simulink model "Sim_Knickarmroboter_AndreasPaul"  (R2024a)
settings: Solver=VariableStepAuto  StartTime=0.0  StopTime=10.0  RelTol=1e-3
values from neighbouring files (symbols this model uses):
  F_s1 = 8.5e-4    (= 0.00085)    [Initialisierung_Kickarmroboter.m]
  F_s2 = 3.2e-4    (= 0.00032)    [Initialisierung_Kickarmroboter.m]
  g = 9.81    [Initialisierung_Kickarmroboter.m]
  I1 = 0.0309    [Initialisierung_Kickarmroboter.m]
  I2 = 0.0045    [Initialisierung_Kickarmroboter.m]
  l1 = 0.16    [Initialisierung_Kickarmroboter.m]
  l2 = 0.128    [Initialisierung_Kickarmroboter.m]
  m1 = 0.1817    [Initialisierung_Kickarmroboter.m]
  m2 = 0.0944    [Initialisierung_Kickarmroboter.m]
  mu_v1 = 3.843e-6    (= 3.843e-06)    [Initialisierung_Kickarmroboter.m]
  mu_v2 = 3.887e-6    (= 3.887e-06)    [Initialisierung_Kickarmroboter.m]
libraries: slpidlib x1
settings Model: Creator=apaul  LastModifiedBy=apaul

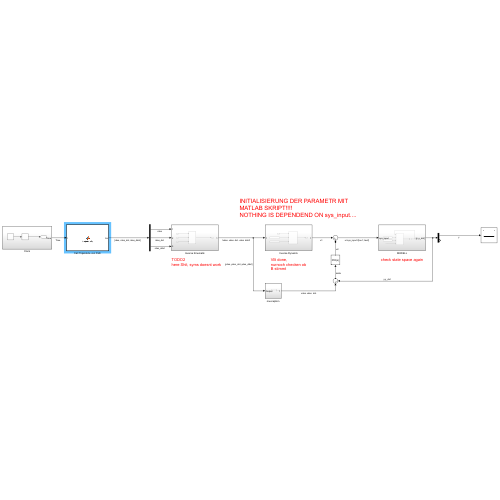
[thumbnail: Simulink's stored preview of the top-level diagram]
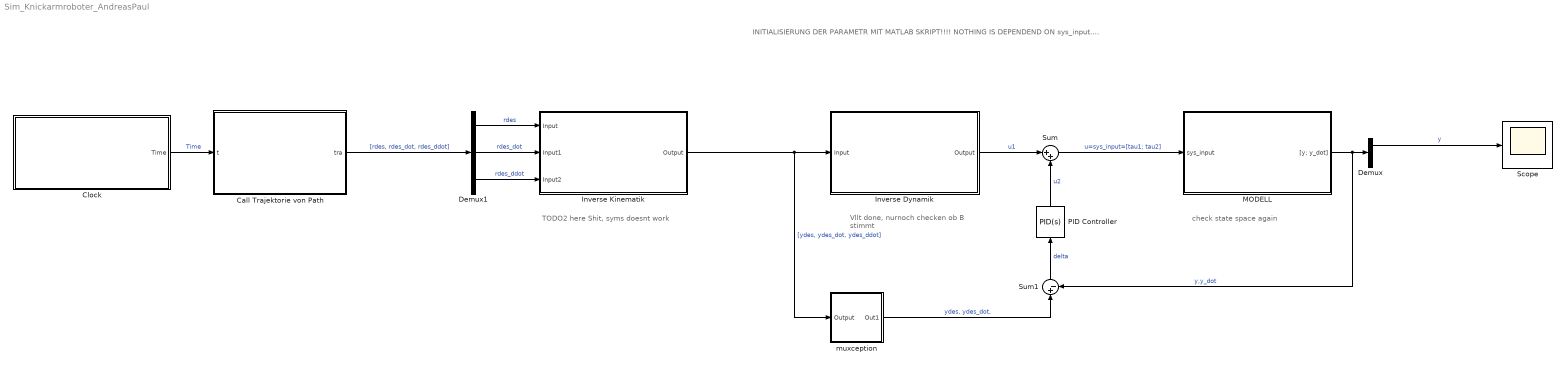
== system Sim_Knickarmroboter_AndreasPaul ==
  note: TODO2
      | here Shit, syms doesnt work
  note: INITIALISIERUNG DER PARAMETR MIT MATLAB SKRIPT!!!!
      | NOTHING IS DEPENDEND ON sys_input....
  note: Vllt done,
      | nurnoch checken ob
      | B stimmt
  note: check state space again
  Call Trajektorie von Path : MATLAB Function  TreatAsAtomicUnit=on
  Clock : Subsystem
  Demux : Demux  Outputs=2
  Demux1 : Demux  Outputs=3
  Inverse Dynamik : Subsystem
  Inverse Kinematik : Subsystem
  MODELL : Subsystem
  PID Controller : slpidlib/PID Controller  Controller=PID  Form=Parallel  TimeDomain=Continuous-time  UseExternalTs=off  SampleTime=-1  IntegratorMethod=Forward Euler  FilterMethod=Forward Euler  ControllerParametersSource=internal  P=1  I=1  UseKiTs=off  D=0  UseExternalDerivativeSource=off  N=100  UseFilter=on  TunerSelectOption=Transfer Function Based (PID Tuner App)  InitialConditionSource=internal  InitialConditionForIntegrator=0  InitialConditionForFilter=0  DifferentiatorICPrevScaledInput=0  ExternalReset=none  TrackingMode=off  Kt=1  LimitOutput=off  SatLimitsSource=internal  UpperSaturationLimit=inf  LowerSaturationLimit=-inf  LinearizeAsGain=on  AntiWindupMode=none  Kb=1  LimitIntegrator=off  UpperIntegratorSaturationLimit=inf  LowerIntegratorSaturationLimit=-inf  POutMin=[]  POutMax=[]  IOutMin=[]  IOutMax=[]  DOutMin=[]  DOutMax=[]  NOutMin=[]  NOutMax=[]  SumOutMin=[]  SumOutMax=[]  SaturationOutMin=[]  SaturationOutMax=[]  PParamMin=[]  PParamMax=[]  IParamMin=[]  IParamMax=[]  DParamMin=[]  DParamMax=[]  NParamMin=[]  NParamMax=[]  KbParamMin=[]  KbParamMax=[]  KtParamMin=[]  KtParamMax=[]  KbOutMin=[]  KbOutMax=[]  KtOutMin=[]  KtOutMax=[]  IntegratorOutMin=[]  IntegratorOutMax=[]  FilterOutMin=[]  FilterOutMax=[]  SumI1OutMin=[]  SumI1OutMax=[]  SumI2OutMin=[]  SumI2OutMax=[]  SumI3OutMin=[]  SumI3OutMax=[]  SumI4OutMin=[]  SumI4OutMax=[]  SumDOutMin=[]  SumDOutMax=[]  DifferentiatorOutMin=[]  DifferentiatorOutMax=[]  FilterDiffOutCoefMin=[]  FilterDiffOutCoefMax=[]  ReciprocalOutMin=[]  ReciprocalOutMax=[]  SumDenOutMin=[]  SumDenOutMax=[]  SumNumOutMin=[]  SumNumOutMax=[]  DivideOutMin=[]  DivideOutMax=[]  UdiffTsProdOutMin=[]  UdiffTsProdOutMax=[]  NTsProdOutMin=[]  NTsProdOutMax=[]  UintegralTsProdOutMin=[]  UintegralTsProdOutMax=[]  UngainTsProdOutMin=[]  UngainTsProdOutMax=[]  ClampingZeroOutDataTypeStr=Inherit: Inherit via back propagation  ClampingZeroOutMin=[]  ClampingZeroOutMax=[]  FilterDenConstantOutDataTypeStr=Inherit: Inherit via back propagation  FilterDenConstantOutMin=[]  FilterDenConstantOutMax=[]  PCopyOutDataTypeStr=Inherit: Inherit via back propagation  PCopyOutMin=[]  PCopyOutMax=[]  NCopyOutDataTypeStr=Inherit: Inherit via back propagation  NCopyOutMin=[]  NCopyOutMax=[]  IntegratorContinuousStateAttributes=''  IntegratorStateMustResolveToSignalObject=off  IntegratorRTWStateStorageClass=Auto  FilterContinuousStateAttributes=''  FilterStateMustResolveToSignalObject=off  FilterRTWStateStorageClass=Auto  ParallelPVariant=InternalParameters  IdealPVariant=Disabled  IVariant=InternalParameters  DVariant=InternalParameters  IntegratorVariant=Continuous  SatVariant=Disabled  AWVariant=Passthrough  PCopyVariant=Disabled  TRVariant=Disabled  FdbkBlocksVariant=Forward  IdealPFdbkVariant=Disabled  SatFdbkVariant=Disabled  DerivativeFilterVariant=ContFilter  NVariant=InternalParameters  NCopyVariant=Disabled  FilterICVariant=InternalICsFilter  IntegratorICVariant=InternalICs  ExternalResetVariant=Disabled  TRSumVariant=Passthrough  SumFdbkVariant=Disabled  SumVariant=Sum_PID  TsampFilterVariant=InternalTs  TsampNgainVariant=Passthrough  TsampIntegralVariant=Disabled_SignalSpec  ExternalSaturationOutDataTypeStr=Inherit: Same as second input  DerivativeSourceVariant=ErrorSignal
  Scope : Scope
  Sum : Sum  Inputs=|++
  Sum1 : Sum  Inputs=|+-
  muxception : Subsystem
  wires:
  Sum/1 -> MODELL/1(sys_input)  "u=sys_input=[tau1; tau2]"
  PID Controller/1 -> Sum/2  "u2"
  Sum1/1 -> PID Controller/1  "delta"
  MODELL/1("[y; y_dot]") -> Sum1/2, Demux/1  "y,y_dot"
  Inverse Kinematik/1(Output) -> Inverse Dynamik/1(Input), muxception/1(Output)  "[ydes, ydes_dot, ydes_ddot]"
  Inverse Dynamik/1(Output) -> Sum/1  "u1"
  Demux/1 -> Scope/1  "y"
  muxception/1(Out1) -> Sum1/1  "ydes, ydes_dot,"
  Call Trajektorie von Path/1(tra) -> Demux1/1  "[rdes, rdes_dot, rdes_ddot]"
  Demux1/3 -> Inverse Kinematik/3(Input2)  "rdes_ddot"
  Demux1/2 -> Inverse Kinematik/2(Input1)  "rdes_dot"
  Demux1/1 -> Inverse Kinematik/1(Input)  "rdes"
  Clock/1(Time) -> Call Trajektorie von Path/1(t)  "Time"

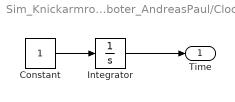
== system Sim_Knickarmroboter_AndreasPaul/Clock ==
  Constant : Constant
  Integrator : Integrator
  Time : Outport
  wires:
  Constant/1 -> Integrator/1
  Integrator/1 -> Time/1

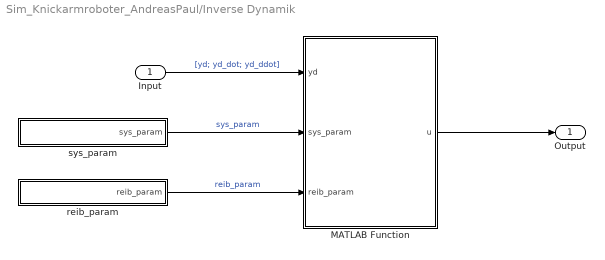
== system Sim_Knickarmroboter_AndreasPaul/Inverse Dynamik ==
  Input : Inport
  MATLAB Function : MATLAB Function  TreatAsAtomicUnit=on
  reib_param : Subsystem
  sys_param : Subsystem
  Output : Outport
  wires:
  Input/1 -> MATLAB Function/1(yd)  "[yd; yd_dot; yd_ddot]"
  MATLAB Function/1(u) -> Output/1
  sys_param/1(sys_param) -> MATLAB Function/2(sys_param)  "sys_param"
  reib_param/1(reib_param) -> MATLAB Function/3(reib_param)  "reib_param"

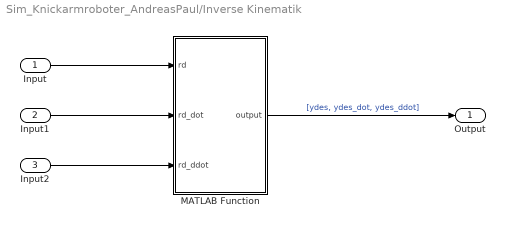
== system Sim_Knickarmroboter_AndreasPaul/Inverse Kinematik ==
  Input : Inport
  Input1 : Inport  Port=2
  Input2 : Inport  Port=3
  MATLAB Function : MATLAB Function  TreatAsAtomicUnit=on
  Output : Outport
  wires:
  Input/1 -> MATLAB Function/1(rd)
  MATLAB Function/1(output) -> Output/1  "[ydes, ydes_dot, ydes_ddot]"
  Input1/1 -> MATLAB Function/2(rd_dot)
  Input2/1 -> MATLAB Function/3(rd_ddot)

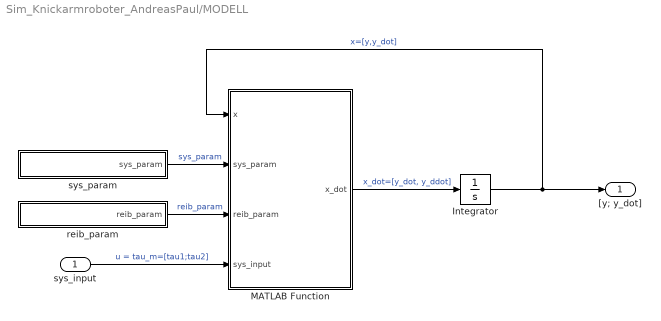
== system Sim_Knickarmroboter_AndreasPaul/MODELL ==
  sys_input : Inport
  Integrator : Integrator
  MATLAB Function : MATLAB Function  TreatAsAtomicUnit=on
  reib_param : Subsystem
  sys_param : Subsystem
  "[y; y_dot]" : Outport
  wires:
  MATLAB Function/1(x_dot) -> Integrator/1  "x_dot=[y_dot, y_ddot]"
  Integrator/1 -> MATLAB Function/1(x), "[y; y_dot]"/1  "x=[y,y_dot]"
  sys_input/1 -> MATLAB Function/4(sys_input)  "u = tau_m=[tau1;tau2]"
  sys_param/1(sys_param) -> MATLAB Function/2(sys_param)  "sys_param"
  reib_param/1(reib_param) -> MATLAB Function/3(reib_param)  "reib_param"

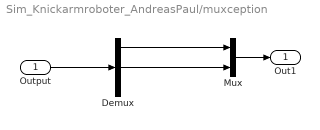
== system Sim_Knickarmroboter_AndreasPaul/muxception ==
  Output : Inport
  Demux : Demux  Outputs=3
  Mux : Mux  Inputs=2
  Out1 : Outport
  wires:
  Output/1 -> Demux/1
  Demux/1 -> Mux/1
  Demux/2 -> Mux/2
  Mux/1 -> Out1/1

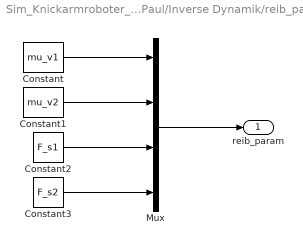
== system Sim_Knickarmroboter_AndreasPaul/Inverse Dynamik/reib_param ==
  Constant : Constant  Value=mu_v1
  Constant1 : Constant  Value=mu_v2
  Constant2 : Constant  Value=F_s1
  Constant3 : Constant  Value=F_s2
  Mux : Mux
  reib_param : Outport
  wires:
  Constant3/1 -> Mux/4
  Constant2/1 -> Mux/3
  Constant1/1 -> Mux/2
  Constant/1 -> Mux/1
  Mux/1 -> reib_param/1

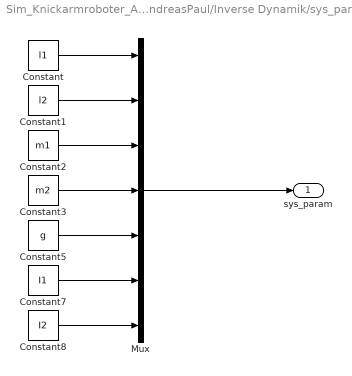
== system Sim_Knickarmroboter_AndreasPaul/Inverse Dynamik/sys_param ==
  Constant : Constant  Value=l1
  Constant1 : Constant  Value=l2
  Constant2 : Constant  Value=m1
  Constant3 : Constant  Value=m2
  Constant5 : Constant  Value=g
  Constant7 : Constant  Value=I1
  Constant8 : Constant  Value=I2
  Mux : Mux  Inputs=7
  sys_param : Outport
  wires:
  Constant8/1 -> Mux/7
  Constant7/1 -> Mux/6
  Constant3/1 -> Mux/4
  Constant2/1 -> Mux/3
  Constant1/1 -> Mux/2
  Constant/1 -> Mux/1
  Mux/1 -> sys_param/1
  Constant5/1 -> Mux/5

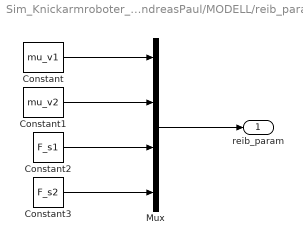
== system Sim_Knickarmroboter_AndreasPaul/MODELL/reib_param ==
  Constant : Constant  Value=mu_v1
  Constant1 : Constant  Value=mu_v2
  Constant2 : Constant  Value=F_s1
  Constant3 : Constant  Value=F_s2
  Mux : Mux
  reib_param : Outport
  wires:
  Constant3/1 -> Mux/4
  Constant2/1 -> Mux/3
  Constant1/1 -> Mux/2
  Constant/1 -> Mux/1
  Mux/1 -> reib_param/1

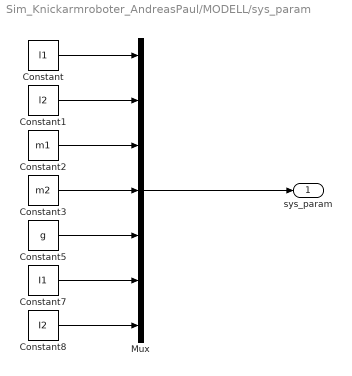
== system Sim_Knickarmroboter_AndreasPaul/MODELL/sys_param ==
  Constant : Constant  Value=l1
  Constant1 : Constant  Value=l2
  Constant2 : Constant  Value=m1
  Constant3 : Constant  Value=m2
  Constant5 : Constant  Value=g
  Constant7 : Constant  Value=I1
  Constant8 : Constant  Value=I2
  Mux : Mux  Inputs=7
  sys_param : Outport
  wires:
  Constant8/1 -> Mux/7
  Constant7/1 -> Mux/6
  Constant3/1 -> Mux/4
  Constant2/1 -> Mux/3
  Constant1/1 -> Mux/2
  Constant/1 -> Mux/1
  Mux/1 -> sys_param/1
  Constant5/1 -> Mux/5

== matlab function Sim_Knickarmroboter_AndreasPaul/Inverse Dynamik/MATLAB Function ==
  data: yd input; u output; sys_param input; reib_param input
function u = fcn(yd, sys_param, reib_param)

%%%%%to be deleted
sys_input = [0; 0];
%%%%%

M = MassMatrix(yd(1:3), sys_param, sys_input);
D = DMatrix(yd(1:3), yd(4:6), sys_param, sys_input, reib_param);
G = GVector(yd(1:3), sys_param, sys_input, reib_param);
tau_R = CALCtau_R(x(1:3), x(4:6), sys_param, sys_input, reib_param);

%B ziemlich sicher einfach nur Identity, da tau_m im y Raum
B = eye(2,2);

u = B \ (M * yd(7:9) + D + G - tau_R);
end

== matlab function Sim_Knickarmroboter_AndreasPaul/MODELL/MATLAB Function ==
  data: x input; sys_param input; reib_param input; x_dot output; sys_input input
function x_dot = fcn(x, sys_param, reib_param, sys_input)
%x(1:3)=y
%x(4:6)=y_dot
M = MassMatrix(x(1:3), sys_param, sys_input);
D = DMatrix(x(1:3), x(4:6), sys_param, sys_input, reib_param);
G = GVector(x(1:3), sys_param, sys_input, reib_param);
tau_R = CALCtau_R(x(1:3), x(4:6), sys_param, sys_input, reib_param);

%State Space System
x_dot = [0, 1;
         0, M \ (tau_R + sys_input - G - D)];
end

== matlab function Sim_Knickarmroboter_AndreasPaul/Inverse Kinematik/MATLAB Function ==
  data: rd input; output output; rd_dot input; rd_ddot input
function output = fcn(rd,rd_dot,rd_ddot)
%SHIT, I don t want to do integration, but technically i could define
%alpha0 beta0 and shit and then compute the numerical shit then integrate
%and ... but annoying
J = Jfunc()


output = [yd; yd_dot; yd_ddot];
end

== matlab function Sim_Knickarmroboter_AndreasPaul/Call Trajektorie von Path ==
  data: tra output; t input
function tra = trajektorie(t)
%Trajektorie
tra = CALCtrajektorie(t);
end
